simulink library "HeatTransfer2Ground_ISO13370"  (Simulink 7.6)
settings: Solver=ode45  StartTime=0.0  StopTime=10.0  RelTol=1e-3
settings Model: Creator=drhf  LastModifiedBy=drhf

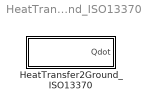
== system HeatTransfer2Ground_ISO13370 ==
  HeatTransfer2Ground_ISO13370 : Subsystem  mask(Heat Transfer to Ground){wallsize=[7 10], gammat=0, Tmeaninside=23.8, deltathetai=3.8, Tmeanoutside=11, deltathetae=9.3, tshift=319*3600, dwall=0.4, cond_ground=2.0, cp_ground=800, rho_ground=2500, rtot=1./0.183}
      mask prompts: wallsize "size of slab [m] [length width]"; gammat "linear thermal transmittance associated with wall/floor junctions [W/mK]"; Tmeaninside "mean inside temperature over one year [°C]"; deltathetai "amplitude of monthly mean internal temperature [°C]"; Tmeanoutside "mean outside temperature over one year [°C]"; deltathetae "amplitude of monthly mean outside temperature [°C]"; tshift "time shift where external temperature sine-curve shows a mimimum [h]"; dwall "average thickness of side walls inlcuding all layers [m]"; cond_ground "conductivity of ground [W/(m*K)]"; cp_ground "capacity of ground [J/(kg*K)]"; rho_ground "density of ground [kg/m^3]"; rtot "total thermal resistance of slab (between Troom and Tground) [m²K/W]"
      mask help: Ground heat transfer for a floor "SLAB ON GROUND" according to ISO 13370:2007.

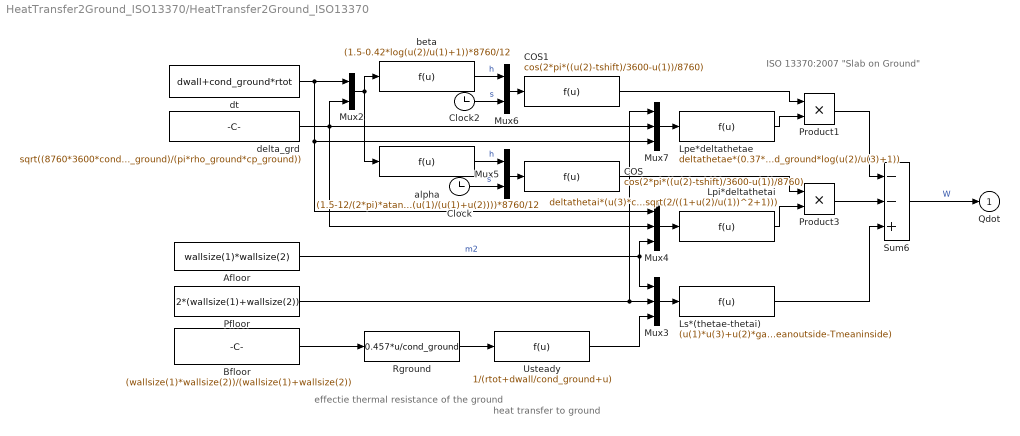
== system HeatTransfer2Ground_ISO13370/HeatTransfer2Ground_ISO13370 ==
  note: ISO 13370:2007 "Slab on Ground"
  note: effectie thermal resistance
      | of the ground
  note: heat transfer
      | to ground
  Afloor : Constant  Value=wallsize(1)*wallsize(2)
  Bfloor : Constant  Value=(wallsize(1)*wallsize(2))/(wallsize(1)+wallsize(2))
  COS : Fcn  Expr=cos(2*pi*((u(2)-tshift)/3600-u(1))/8760)
  COS1 : Fcn  Expr=cos(2*pi*((u(2)-tshift)/3600-u(1))/8760)
  Clock : Clock
      settings: Decimation=10
  Clock2 : Clock
      settings: Decimation=10
  Lpe*deltathetae : Fcn  Expr=deltathetae*(0.37*u(1)*cond_ground*log(u(2)/u(3)+1))
  Lpi*deltathetai : Fcn  Expr=deltathetai*(u(3)*cond_ground/u(1)*sqrt(2/((1+u(2)/u(1))^2+1)))
  Ls*(thetae-thetai) : Fcn  Expr=(u(1)*u(3)+u(2)*gammat)*(Tmeanoutside-Tmeaninside)
  Mux2 : Mux  Inputs=2
  Mux3 : Mux  Inputs=3
  Mux4 : Mux  Inputs=3
  Mux5 : Mux  Inputs=2
  Mux6 : Mux  Inputs=2
  Mux7 : Mux  Inputs=3
  Pfloor : Constant  Value=2*(wallsize(1)+wallsize(2))
  Product1 : Product  SaturateOnIntegerOverflow=on  RndMeth=Zero  InputSameDT=on  OutDataTypeStr=Inherit: Same as first input
  Product3 : Product  SaturateOnIntegerOverflow=on  RndMeth=Zero  InputSameDT=on  OutDataTypeStr=Inherit: Same as first input
  Rground : Fcn  Expr=0.457*u/cond_ground
  Sum6 : Sum  Inputs=--+
  Usteady : Fcn  Expr=1/(rtot+dwall/cond_ground+u)
  alpha : Fcn  Expr=(1.5-12/(2*pi)*atan(u(1)/(u(1)+u(2))))*8760/12
  beta : Fcn  Expr=(1.5-0.42*log(u(2)/u(1)+1))*8760/12
  delta_grd : Constant  Value=sqrt((8760*3600*cond_ground)/(pi*rho_ground*cp_ground))
  dt : Constant  Value=dwall+cond_ground*rtot
  Qdot : Outport  InitialOutput=0
  wires:
  Sum6/1 -> Qdot/1  "W"
  Mux7/1 -> Lpe*deltathetae/1
  Product1/1 -> Sum6/1
  Lpe*deltathetae/1 -> Product1/2
  COS1/1 -> Product1/1
  Mux6/1 -> COS1/1
  Clock2/1 -> Mux6/2  "s"
  beta/1 -> Mux6/1  "h"
  Ls*(thetae-thetai)/1 -> Sum6/3
  Product3/1 -> Sum6/2
  COS/1 -> Product3/1
  Mux5/1 -> COS/1
  Clock/1 -> Mux5/2  "s"
  alpha/1 -> Mux5/1  "h"
  Lpi*deltathetai/1 -> Product3/2
  Mux4/1 -> Lpi*deltathetai/1
  Usteady/1 -> Mux3/3
  Pfloor/1 -> Mux7/1, Mux3/2
  Afloor/1 -> Mux3/1, Mux4/3  "m2"
  Mux3/1 -> Ls*(thetae-thetai)/1
  Mux2/1 -> beta/1, alpha/1
  delta_grd/1 -> Mux2/2, Mux7/2, Mux4/2
  dt/1 -> Mux7/3, Mux4/1, Mux2/1
  Bfloor/1 -> Rground/1
  Rground/1 -> Usteady/1
